simulink model "Manuf30_M6"  (R2023a)
settings: Solver=FixedStepAuto  StartTime=0.0  StopTime=720  FixedStep=1  RelTol=1e-3
model workspace (MAT data in the model file):
  EPdefault = 5
  EPmax = 5
  FRm = 120
  IPdefault = 5
libraries: simulink x25
(part 2 of 2)

== stateflow chart Manuf30_M6/State Transition Table5 ==
  state Init
    T=0;
    Warehouse=1;
    Damage=0;
    Inventory=1;
  state Great
    Warehouse=0;
    RT=90;
    T=T+1;
  state Major
    Warehouse=0;
    RT=45;
    T=T+1;
  state Strong
    Warehouse=0
    RT=10;
    T=T+1;
  state Moderate
    Warehouse=0;
    RT=1;
    T=T+1;
  state Over
    Warehouse=1;
  (default) -> Init
  Init -> (junction 29) [order 3] : [Magnitude>=7]
      | {Inventory=0.5; Damage=1}
  (junction 29) -> (junction 23)
  Init -> (junction 41) [order 4] : [Magnitude>=6]
      | {Inventory=0.9}
  (junction 41) -> (junction 39)
  Init -> (junction 157) [order 5] : [Magnitude>=5]
  (junction 157) -> (junction 165)
  Init -> (junction 165) [order 1] : [Magnitude>0 & Reinforcement==1]
  (junction 165) -> (junction 32)
  Init -> Great [order 2] : [Magnitude>=8]
      | {Inventory=0.2; Damage=2}
  Great -> (junction 175) : [T>=RT]
  (junction 175) -> (junction 172)
  (junction 23) -> Major
  Major -> (junction 172) : [T>=RT]
  (junction 172) -> (junction 169)
  (junction 39) -> Strong
  Strong -> (junction 169) : [T>=RT]
  (junction 169) -> (junction 132)
  (junction 32) -> Moderate
  Moderate -> Over : [T>=RT]
  (junction 132) -> Over
  data: Magnitude input; T local; RT local; Warehouse output; Inventory output; Damage output; Reinforcement input

== stateflow chart Manuf30_M6/State Transition Table6 ==
  state Init
    T=0;
    LogisticsCenter=1;
    Damage=0;
  state Great
    LogisticsCenter=0;
    RT=90;
    T=T+1;
  state Major
    LogisticsCenter=0;
    RT=45;
    T=T+1;
  state Strong
    LogisticsCenter=0
    RT=10;
    T=T+1;
  state Moderate
    LogisticsCenter=0;
    RT=1;
    T=T+1;
  state Over
    LogisticsCenter=1;
  (default) -> Init
  Init -> (junction 29) [order 3] : [Magnitude>=7]
      | {Damage=1}
  (junction 29) -> (junction 23)
  Init -> (junction 41) [order 4] : [Magnitude>=6]
  (junction 41) -> (junction 39)
  Init -> (junction 153) [order 5] : [Magnitude>=5]
  (junction 153) -> (junction 161)
  Init -> (junction 161) [order 1] : [Magnitude>0 & Reinforcement==1]
  (junction 161) -> (junction 32)
  Init -> Great [order 2] : [Magnitude>=8]
      | {Damage=3}
  Great -> (junction 171) : [T>=RT]
  (junction 171) -> (junction 168)
  (junction 23) -> Major
  Major -> (junction 168) : [T>=RT]
  (junction 168) -> (junction 165)
  (junction 39) -> Strong
  Strong -> (junction 165) : [T>=RT]
  (junction 165) -> (junction 132)
  (junction 32) -> Moderate
  Moderate -> Over : [T>=RT]
  (junction 132) -> Over
  data: Magnitude input; T local; RT local; LogisticsCenter output; Damage output; Reinforcement input
